simulink model "Week2_Sum3"  (R2020b)
settings: Solver=VariableStepAuto  StartTime=0.0  StopTime=120  RelTol=1e-3
PreLoadFcn:
  | clear all;
  | close all;
  | clc;
  | m=1000;
  | b=50;
  | u=500;
settings Model: Creator=Aradhana desai  LastModifiedBy=Aradhana desai

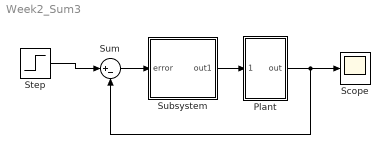
== system Week2_Sum3 ==
  Plant : Subsystem
  Scope : Scope
  Step : Step  Time=0  After=u  SampleTime=0
  Subsystem : Subsystem
  Sum : Sum  Inputs=|+-
  wires:
  Subsystem/1(out1) -> Plant/1(1)
  Step/1 -> Sum/1
  Plant/1(out) -> Sum/2, Scope/1
  Sum/1 -> Subsystem/1(error)

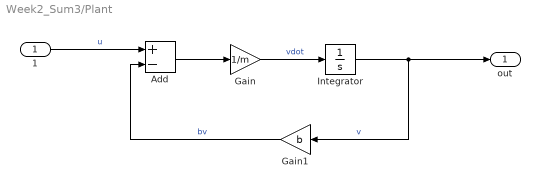
== system Week2_Sum3/Plant ==
  1 : Inport
  Add : Sum  Inputs=+-
  Gain : Gain  Gain=1/m
  Gain1 : Gain  Gain=b
  Integrator : Integrator
  out : Outport
  wires:
  Gain/1 -> Integrator/1  "vdot"
  Integrator/1 -> out/1, Gain1/1  "v"
  Gain1/1 -> Add/2  "bv"
  Add/1 -> Gain/1
  1/1 -> Add/1  "u"

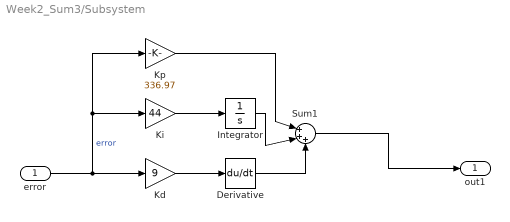
== system Week2_Sum3/Subsystem ==
  error : Inport  OutDataTypeStr=double  PortDimensions=1  SampleTime=0
  Derivative : Derivative
  Integrator : Integrator
  Kd : Gain  Gain=9
  Ki : Gain  Gain=44
  Kp : Gain  Gain=336.97
  Sum1 : Sum  Inputs=|+++
  out1 : Outport  OutDataTypeStr=double  PortDimensions=1  SampleTime=0
  wires:
  Kd/1 -> Derivative/1
  Ki/1 -> Integrator/1
  error/1 -> Kd/1, Ki/1, Kp/1  "error"
  Derivative/1 -> Sum1/3
  Sum1/1 -> out1/1
  Kp/1 -> Sum1/1
  Integrator/1 -> Sum1/2
